simulink subsystem "EgoState"  (R2024b)
settings: Solver=VariableStepAuto  StartTime=0.0  StopTime=10.0  RelTol=1e-3
settings Model: Creator=Tong  LastModifiedBy=Tong

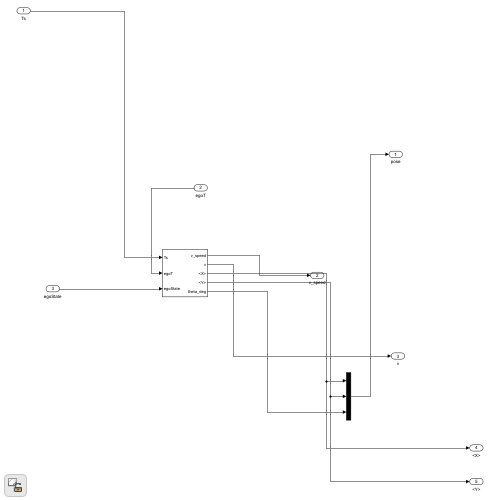
[thumbnail: Simulink's stored preview of the top-level diagram]
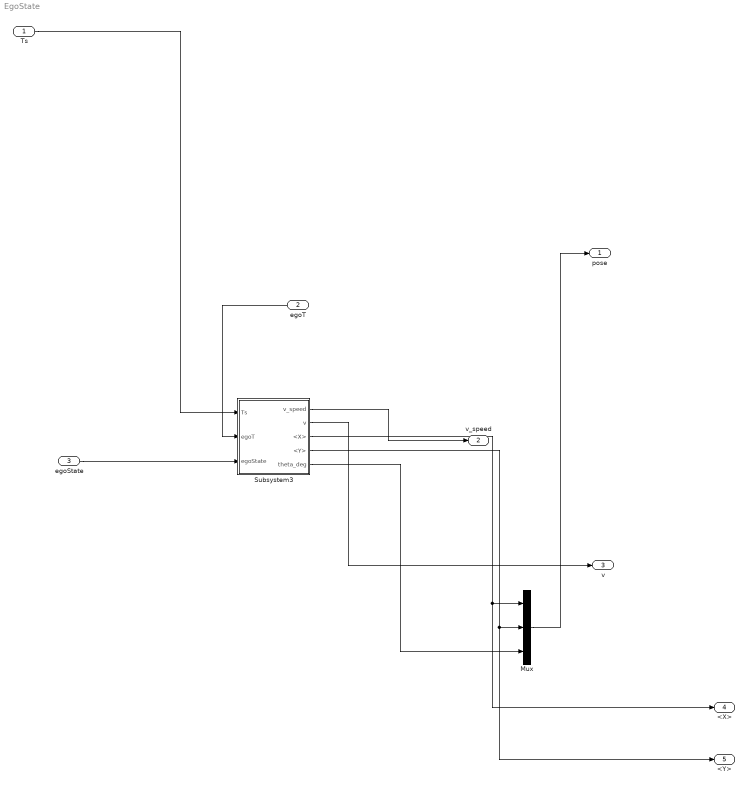
== system EgoState ==
  Ts : Inport
  egoT : Inport  Port=2
  egoState : Inport  Port=3
  Mux : Mux  Inputs=3
  Subsystem3 : Subsystem
  pose : Outport
  v_speed : Outport  Port=2
  v : Outport  Port=3
  <X> : Outport  Port=4
  <Y> : Outport  Port=5
  wires:
  Subsystem3/3(<X>) -> Mux/1, <X>/1
  Ts/1 -> Subsystem3/1(Ts)
  Mux/1 -> pose/1
  Subsystem3/4(<Y>) -> Mux/2, <Y>/1
  egoT/1 -> Subsystem3/2(egoT)
  Subsystem3/2(v) -> v/1
  Subsystem3/5(theta_deg) -> Mux/3
  egoState/1 -> Subsystem3/3(egoState)
  Subsystem3/1(v_speed) -> v_speed/1

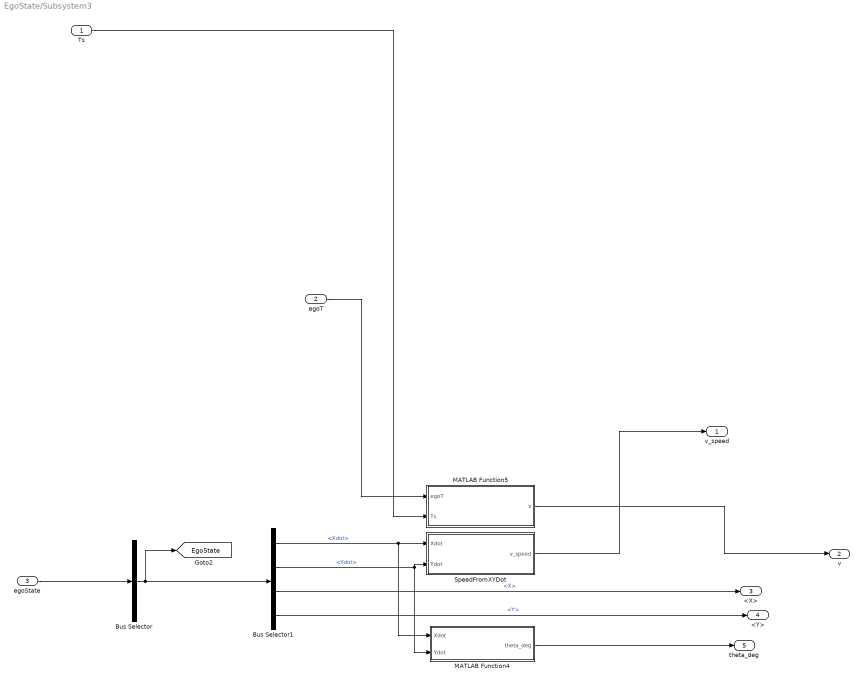
== system EgoState/Subsystem3 ==
  Ts : Inport
  egoT : Inport  Port=2
  egoState : Inport  Port=3
  Bus Selector : BusSelector  OutputSignals=Body.InertFrm.Cg.Disp.X,Body.InertFrm.Cg.Disp.Y,Body.InertFrm.Cg.Disp.Z,Body.InertFrm.Cg.Ang.phi,Body.InertFrm.Cg.Ang.theta,Body.InertFrm.Cg.Ang.psi,Body.InertFrm.Cg.Vel.Xdot,Body.InertFrm.Cg.Vel.Ydot,Body.InertFrm.Cg.Vel.Zdot  OutputAsBus=on
  Bus Selector1 : BusSelector  OutputSignals=Xdot,Ydot,X,Y
  MATLAB Function4 : MATLAB Function  TreatAsAtomicUnit=on
  MATLAB Function5 : MATLAB Function  TreatAsAtomicUnit=on
  SpeedFromXYDot : MATLAB Function  TreatAsAtomicUnit=on
  v_speed : Outport
  v : Outport  Port=2
  <X> : Outport  Port=3
  <Y> : Outport  Port=4
  theta_deg : Outport  Port=5
  tag scope: EgoState=global
  wires:
  SpeedFromXYDot/1(v_speed) -> v_speed/1
  egoT/1 -> MATLAB Function5/1(egoT)
  Ts/1 -> MATLAB Function5/2(Ts)
  MATLAB Function5/1(v) -> v/1
  Bus Selector1/4 -> <Y>/1  "<Y>"
  MATLAB Function4/1(theta_deg) -> theta_deg/1
  egoState/1 -> Bus Selector/1
  Bus Selector1/1 -> SpeedFromXYDot/1(Xdot), MATLAB Function4/1(Xdot)  "<Xdot>"
  Bus Selector/1 -> [EgoState], Bus Selector1/1
  Bus Selector1/3 -> <X>/1  "<X>"
  Bus Selector1/2 -> SpeedFromXYDot/2(Ydot), MATLAB Function4/2(Ydot)  "<Ydot>"

== matlab function EgoState/Subsystem3/SpeedFromXYDot ==
  data: Xdot input; v_speed output; Ydot input
function v_speed = SpeedFromXYDot(Xdot, Ydot)
%#codegen
% SpeedFromXYDot 由世界坐标速度分量计算车速大小（m/s）
%
% 输入:
%   Xdot, Ydot - 世界坐标系速度分量 (m/s)，可正可负
% 输出:
%   v_speed    - 车速大小 (m/s)，非负

v_speed = sqrt(Xdot*Xdot + Ydot*Ydot);

% 防止数值误差导致出现极小负值（理论上不会，但更稳）
if v_speed < 0
    v_speed = 0;
end
end

== matlab function EgoState/Subsystem3/MATLAB Function4 ==
  settings: updateMethod=DISCRETE
  data: Xdot input; theta_deg output; Ydot input

% function theta_deg = HeadingFromXYDot(Xdot, Ydot)
% %#codegen
% persistent theta_last
% if isempty(theta_last)
%     theta_last = 0;
% end
% 
% v = sqrt(Xdot*Xdot + Ydot*Ydot);
% 
% if v < 0.2
%     % 低速/接近静止：保持上一次航向，避免乱跳
%     theta_deg = theta_last;
% else
%     theta_deg = atan2d(Ydot, Xdot);
%     % wrap到[-180,180]
%     while theta_deg > 180,  theta_deg = theta_deg - 360; end
%     while theta_deg < -180, theta_deg = theta_deg + 360; end
%     theta_last = theta_deg;
% end
% end

function theta_deg = HeadingFromXYDot(Xdot, Ydot)
%#codegen
theta_deg = atan2d(Ydot, Xdot);

% wrap到[-180,180]，避免跳变
while theta_deg > 180
    theta_deg = theta_deg - 360;
end
while theta_deg < -180
    theta_deg = theta_deg + 360;
end
end


% function theta_deg = HeadingFromXYDot_Stable(Xdot, Ydot)
% %#codegen
% Ts = 0.05;          % 按你的控制采样时间改
% v_hold = 1;       % 低于该速度不更新航向（0.4~1.0都可）
% maxYawRate = 120;   % deg/s 航向变化率限幅（60~180可调）
% alpha = 0.85;       % 角度滤波（越大越平滑）
% 
% persistent theta_filt init
% if isempty(init)
%     theta_filt = 0;
%     init = true;
% end
% 
% v = hypot(Xdot, Ydot);
% 
% % 速度方向航向
% theta_meas = atan2d(Ydot, Xdot);
% theta_meas = wrapTo180(theta_meas);
% 
% % 低速保持：不更新测量
% if v < v_hold
%     theta_deg = theta_filt;
%     return;
% end
% 
% % 角度差（考虑wrap）
% e = wrapTo180(theta_meas - theta_filt);
% 
% % 角速度限幅（防瞬跳）
% maxStep = maxYawRate * Ts;
% if e >  maxStep, e =  maxStep; end
% if e < -maxStep, e = -maxStep; end
% 
% % 一阶滤波（在角度差上滤）
% theta_filt = wrapTo180(theta_filt + (1-alpha)*e);
% 
% theta_deg = theta_filt;
% end
% 
% function y = wrapTo180(x)
% y = mod(x+180, 360) - 180;
% end


% function theta_deg = HeadingFromXYDot_Stable(Xdot, Ydot)
% %#codegen
% Ts = 0.05;          % 按你的控制采样时间改
% v_hold = 1.0;       % 低于该速度不更新航向（0.4~1.0都可）
% maxYawRate = 120;   % deg/s 航向变化率限幅（60~180可调）
% alpha = 0.85;       % 角度滤波系数（越大越平滑，0~1）
% 
% persistent theta_filt yawInit
% if isempty(theta_filt)
%     theta_filt = 0;
%     yawInit = false;
% end
% 
% v = hypot(Xdot, Ydot);
% 
% % 低速保持：不更新测量，直接返回上一次滤波值
% if v < v_hold
%     theta_deg = theta_filt;
%     return;
% end
% 
% % 高速时，计算速度方向航向
% theta_meas = atan2d(Ydot, Xdot);
% theta_meas = wrapTo180(theta_meas);
% 
% % 首次有效速度：直接赋值，防止从0度跳到真实航向
% if ~yawInit
%     theta_filt = theta_meas;
%     yawInit = true;
% end
% 
% % 角度差（考虑wrap）
% e = wrapTo180(theta_meas - theta_filt);
% 
% % 角速度限幅（防瞬跳）
% maxStep = maxYawRate * Ts;
% if e >  maxStep, e =  maxStep; end
% if e < -maxStep, e = -maxStep; end
% 
% % 一阶滤波（在受限误差上滤）
% theta_filt = wrapTo180(theta_filt + (1-alpha)*e);
% 
% theta_deg = theta_filt;
% end
% 
% function y = wrapTo180(x)
% y = mod(x+180, 360) - 180;
% end

== matlab function EgoState/Subsystem3/MATLAB Function5 ==
  data: egoT input; v output; Ts input
function v = SpeedFromUEPos(egoT, Ts)
%#codegen
persistent prev init
if isempty(init)
    prev = egoT(1:2);
    init = true;
end
vxy = (egoT(1:2) - prev)/Ts;
prev = egoT(1:2);
v = hypot(vxy(1), vxy(2));
end
